simulink model "sampleModel1701"  (R2023a)
settings: Solver=VariableStepAuto  StartTime=0.0  StopTime=10.0  RelTol=1e-3
libraries: hdlsllib x3, simulink x1
settings Model: Creator=user1  LastModifiedBy=user1

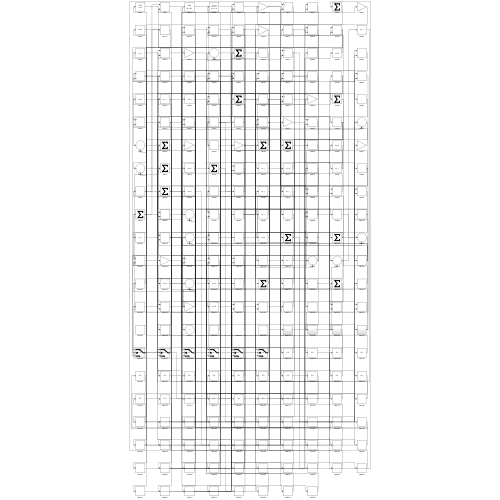
[thumbnail: Simulink's stored preview of the top-level diagram]
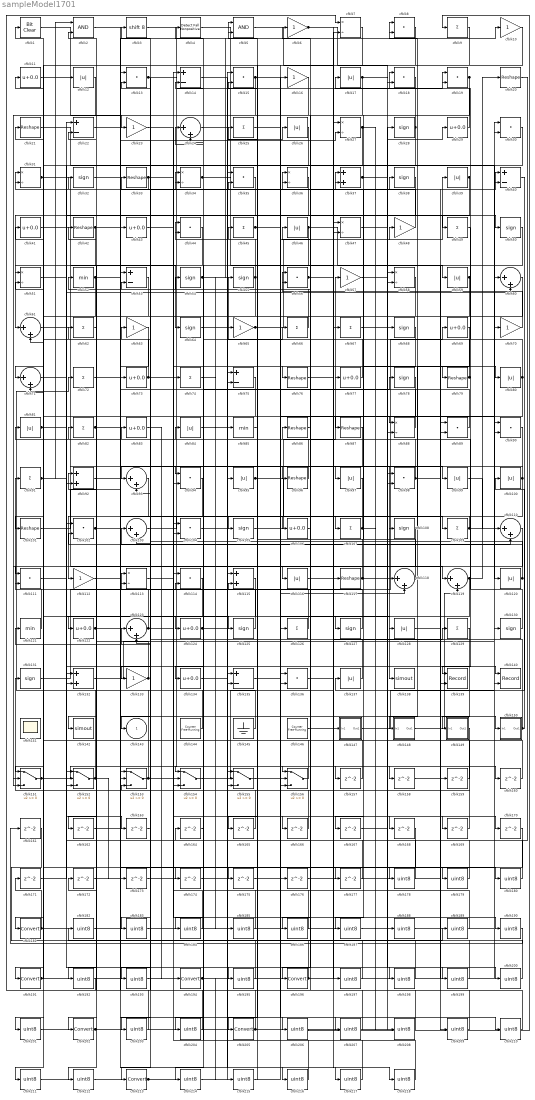
== system sampleModel1701 ==
  cfblk1 : simulink/Logic and Bit Operations/Bit Clear  iBit=0
      settings: LibrarySourceBlock=|
      | hdlsllib/Logic and Bit
      | Operations/Bit Clear
  cfblk{6,10,16,23,48,57,63,65,70,112,133} (11 alike) : Gain
  cfblk{12,17,26,39,46,59,80..81,84,95,97,99..100,116,120,128,137} (17 alike) : Abs  SaturateOnIntegerOverflow=off
  cfblk{20..21,33,42,76,79,86..87,96,101,117} (11 alike) : Reshape
  cfblk{8,13,15,18..19,30,35,44,56,89..90,94,98,102,104,111,114,136} (18 alike) : DotProduct  OutDataTypeStr=Inherit: Inherit via internal rule
  cfblk{24,60..61,71,93,103,110,118..119,123} (10 alike) : Sum  Inputs=|++
  cfblk{28,32,38,50,54..55,64,68,78,105,108,125,127,130..131} (15 alike) : Signum
  cfblk{11,29,41,43,69,73,77,83,106,122,124,134} (12 alike) : Bias  Bias=0.0  SaturateOnIntegerOverflow=off
  cfblk{9,25,45,49,62,66..67,72,74,82,91,107,109,126,129} (15 alike) : Sum  Inputs=+
  cfblk{7,27,31,34,36,47,51,58,88,113} (10 alike) : Product  Inputs=*/  RndMeth=Zero  SaturateOnIntegerOverflow=on
  cfblk{37,92,115,132} (4 alike) : Sum
  cfblk121 : MinMax
  cfblk{14,22,40,53,75,135} (6 alike) : Sum  Inputs=+-
  cfblk138 : ToWorkspace  VariableName=simout  SaveFormat=Timeseries  SampleTime=-1
  cfblk139 : Record  FileSettingsInternal="{\"entries\":[{\"content\":{\"excelSettings\":{\"content\":{},\"type\":\"Streamout.ExcelSettings\"}},\"type\":\"Streamout.FileSettingStorage\",\"uuid\":\"\"}],\"packageUris\":[\"http:\\/\\/schema.mathworks.com\\/mf0\\/streamout_blocks\\/R2020a\"],\"version\":\"1.0\"}"  Layout=[1 1]  SignalsInternal="{\"entries\":[{\"content\":{\"signals\":[{\"content\":{\"blockPath\":[],\"dimensions\":[1],\"domain\":\"\",\"lineColor\":\"#a2142f\",\"plots\":[1],\"port\":1,\"signalID\":3074,\"signalName\":\"XY Graph:1\"},\"type\":\"RecordBlkView.Signal\",\"uuid\":\"\"},{\"content\":{\"blockPath\":[],\"dimensions\":[1],\"domain\":\"\",\"lineColor\":\"#139fff\",\"plots\":[1],\"port\":2,\"signalID\":3077,\"signalName\":\"XY Graph:2\"},\"type\":\"RecordBlkView.Signal\",\"uuid\":\"\"}]},\"type\":\"RecordBlkView.InputSignals\",\"uuid\":\"\"}],\"packageUris\":[\"http:\\/\\/schema.mathworks.com\\/mf0\\/streamout_blocks\\/R2020a\"],\"version\":\"1.0\"}"  VisualizationBindings="{\"xyplotplugin\":{\"info\":[{\"series\":[{\"bindingParametersList\":[{\"parameter\":\"X-Axis\",\"signalID\":3074,\"signalName\":\"XY Graph:1\"},{\"parameter\":\"Y-Axis\",\"signalID\":3077,\"signalName\":\"XY Graph:2\"}],\"seriesID\":48839}],\"subplotID\":1}]}}"  CompatibilityTag=XY  st=-1
  cfblk140 : Record  FileSettingsInternal="{\"entries\":[{\"content\":{\"excelSettings\":{\"content\":{},\"type\":\"Streamout.ExcelSettings\"}},\"type\":\"Streamout.FileSettingStorage\",\"uuid\":\"\"}],\"packageUris\":[\"http:\\/\\/schema.mathworks.com\\/mf0\\/streamout_blocks\\/R2020a\"],\"version\":\"1.0\"}"  Layout=[1 1]  SignalsInternal="{\"entries\":[{\"content\":{\"signals\":[{\"content\":{\"blockPath\":[],\"dimensions\":[1],\"domain\":\"\",\"lineColor\":\"#a2142f\",\"plots\":[1],\"port\":1,\"signalID\":3082,\"signalName\":\"XY Graph:1\"},\"type\":\"RecordBlkView.Signal\",\"uuid\":\"\"},{\"content\":{\"blockPath\":[],\"dimensions\":[1],\"domain\":\"\",\"lineColor\":\"#139fff\",\"plots\":[1],\"port\":2,\"signalID\":3085,\"signalName\":\"XY Graph:2\"},\"type\":\"RecordBlkView.Signal\",\"uuid\":\"\"}]},\"type\":\"RecordBlkView.InputSignals\",\"uuid\":\"\"}],\"packageUris\":[\"http:\\/\\/schema.mathworks.com\\/mf0\\/streamout_blocks\\/R2020a\"],\"version\":\"1.0\"}"  VisualizationBindings="{\"xyplotplugin\":{\"info\":[{\"series\":[{\"bindingParametersList\":[{\"parameter\":\"X-Axis\",\"signalID\":3082,\"signalName\":\"XY Graph:1\"},{\"parameter\":\"Y-Axis\",\"signalID\":3085,\"signalName\":\"XY Graph:2\"}],\"seriesID\":35612}],\"subplotID\":1}]}}"  CompatibilityTag=XY  st=-1
  cfblk141 : Scope
      settings: Floating=on
  cfblk142 : ToWorkspace  VariableName=simout  SaveFormat=Timeseries  SampleTime=-1
  cfblk144 : hdlsllib/Sources/Counter Free-Running  NumBits=16  tsamp=-1
  cfblk145 : Ground
  cfblk146 : hdlsllib/Sources/Counter Free-Running  NumBits=16  tsamp=-1
  cfblk147 : Subsystem
      settings: LibrarySourceBlock=|
      | hdlsllib/Ports &
      | Subsystems/Subsystem
  cfblk148 : Subsystem
      settings: LibrarySourceBlock=|
      | hdlsllib/Ports &
      | Subsystems/Subsystem
  cfblk149 : Subsystem
      settings: LibrarySourceBlock=|
      | hdlsllib/Ports &
      | Subsystems/Subsystem
  cfblk150 : Subsystem
      settings: LibrarySourceBlock=|
      | hdlsllib/Ports &
      | Subsystems/Subsystem
  cfblk{151..156} (6 alike) : Switch  SaturateOnIntegerOverflow=off  InputSameDT=off
  cfblk{157..177} (21 alike) : Delay  SampleTime=1
  cfblk{178..180,182..190,192..193,195,197..201,203..204,206..212,214..218} (34 alike) : DataTypeConversion  OutDataTypeStr=uint8  SaturateOnIntegerOverflow=off  RndMeth=Floor
  cfblk{181,191,194,196,202,205,213} (7 alike) : DataTypeConversion  SaturateOnIntegerOverflow=off  RndMeth=Floor
  cfblk2 : Logic  AllPortsSameDT=off  OutDataTypeStr=boolean
  cfblk3 : ArithShift  BitShiftNumber=8
  cfblk4 : hdlsllib/Logic and Bit Operations/Detect Fall Nonpositive  vinit=0  OutDataTypeStr=boolean
  cfblk5 : Logic  AllPortsSameDT=off  OutDataTypeStr=boolean
  cfblk52 : MinMax
  cfblk85 : MinMax
  cfblk143 : Outport  VectorParamsAs1DForOutWhenUnconnected=off
  wires:
  cfblk79/1 -> cfblk55/1, cfblk8/1
  cfblk93/1 -> cfblk112/1
  cfblk74/1 -> cfblk85/1
  cfblk61/1 -> cfblk138/1
  cfblk99/1 -> cfblk110/1
  cfblk3/1 -> cfblk156/1
  cfblk80/1 -> cfblk17/1, cfblk94/1, cfblk212/1
  cfblk41/1 -> cfblk119/1
  cfblk130/1 -> cfblk84/1
  cfblk144/1 -> cfblk92/1
  cfblk54/1 -> cfblk10/1, cfblk76/1, cfblk185/1
  cfblk9/1 -> cfblk205/1
  cfblk40/1 -> cfblk137/1
  cfblk131/1 -> cfblk69/1
  cfblk36/1 -> cfblk61/1
  cfblk137/1 -> cfblk34/1
  cfblk85/1 -> cfblk5/1
  cfblk105/1 -> cfblk57/1
  cfblk152/1 -> cfblk72/1, cfblk173/1
  cfblk5/1 -> cfblk117/1
  cfblk88/1 -> cfblk77/1
  cfblk100/1 -> cfblk93/1, cfblk175/1
  cfblk133/1 -> cfblk62/1, cfblk121/1
  cfblk28/1 -> cfblk23/1, cfblk111/1
  cfblk149/1(Out1) -> cfblk131/1
  cfblk76/1 -> cfblk38/1
  cfblk50/1 -> cfblk134/1
  cfblk56/1 -> cfblk116/1, cfblk88/2
  cfblk145/1 -> cfblk21/1
  cfblk150/1(Out1) -> cfblk33/1, cfblk100/1
  cfblk146/1 -> cfblk147/1(In1)
  cfblk124/1 -> cfblk44/1, cfblk166/1
  cfblk33/1 -> cfblk31/2, cfblk35/2, cfblk203/1
  cfblk108/1 -> cfblk18/1, cfblk151/3
  cfblk101/1 -> cfblk36/1
  cfblk87/1 -> cfblk143/1
  cfblk147/1(Out1) -> cfblk119/2
  cfblk59/1 -> cfblk98/2, cfblk167/1, cfblk184/1
  cfblk91/1 -> cfblk41/1, cfblk12/1, cfblk60/2
  cfblk107/1 -> cfblk106/1, cfblk188/1
  cfblk92/1 -> cfblk78/1
  cfblk6/1 -> cfblk58/1, cfblk218/1
  cfblk153/1 -> cfblk52/1, cfblk177/1
  cfblk151/1 -> cfblk154/1, cfblk163/1
  cfblk103/1 -> cfblk108/1
  cfblk117/1 -> cfblk28/1, cfblk45/1
  cfblk125/1 -> cfblk113/1
  cfblk119/1 -> cfblk151/1, cfblk20/1
  cfblk35/1 -> cfblk75/2
  cfblk94/1 -> cfblk122/1
  cfblk31/1 -> cfblk64/1, cfblk49/1
  cfblk1/1 -> cfblk73/1
  cfblk111/1 -> cfblk140/1
  cfblk126/1 -> cfblk32/1
  cfblk98/1 -> cfblk11/1, cfblk170/1
  cfblk10/1 -> cfblk156/2
  cfblk48/1 -> cfblk3/1
  cfblk21/1 -> cfblk120/1
  cfblk49/1 -> cfblk139/1
  cfblk136/1 -> cfblk129/1
  cfblk4/1 -> cfblk67/1
  cfblk132/1 -> cfblk70/1
  cfblk123/1 -> cfblk81/1, cfblk190/1
  cfblk32/1 -> cfblk105/1
  cfblk122/1 -> cfblk5/2, cfblk8/2
  cfblk26/1 -> cfblk93/2
  cfblk16/1 -> cfblk181/1
  cfblk148/1(Out1) -> cfblk130/1
  cfblk156/1 -> cfblk113/2
  cfblk38/1 -> cfblk92/2
  cfblk7/1 -> cfblk191/1
  cfblk115/1 -> cfblk213/1
  cfblk65/1 -> cfblk39/1, cfblk88/1
  cfblk77/1 -> cfblk34/2
  cfblk52/1 -> cfblk27/2, cfblk61/2
  cfblk29/1 -> cfblk19/1
  cfblk43/1 -> cfblk74/1
  cfblk47/1 -> cfblk68/1
  cfblk83/1 -> cfblk194/1
  cfblk73/1 -> cfblk79/1, cfblk51/2
  cfblk34/1 -> cfblk50/1, cfblk126/1
  cfblk128/1 -> cfblk40/1
  cfblk129/1 -> cfblk149/1(In1)
  cfblk42/1 -> cfblk71/1, cfblk199/1
  cfblk12/1 -> cfblk71/2
  cfblk58/1 -> cfblk97/1
  cfblk55/1 -> cfblk132/2, cfblk44/2
  cfblk46/1 -> cfblk139/2, cfblk152/3, cfblk90/2, cfblk154/3
  cfblk39/1 -> cfblk103/2, cfblk51/1
  cfblk112/1 -> cfblk136/2
  cfblk51/1 -> cfblk102/1
  cfblk69/1 -> cfblk148/1(In1)
  cfblk109/1 -> cfblk60/1, cfblk107/1
  cfblk45/1 -> cfblk128/1, cfblk40/2
  cfblk13/1 -> cfblk19/2, cfblk123/2
  cfblk11/1 -> cfblk43/1
  cfblk81/1 -> cfblk2/1, cfblk195/1
  cfblk71/1 -> cfblk125/1
  cfblk64/1 -> cfblk99/1
  cfblk37/1 -> cfblk29/1, cfblk59/1
  cfblk154/1 -> cfblk47/2
  cfblk78/1 -> cfblk127/1
  cfblk70/1 -> cfblk56/1
  cfblk66/1 -> cfblk42/1
  cfblk27/1 -> cfblk152/2, cfblk208/1
  cfblk104/1 -> cfblk66/1
  cfblk120/1 -> cfblk31/1, cfblk82/1, cfblk102/2
  cfblk110/1 -> cfblk142/1
  cfblk18/1 -> cfblk133/1
  cfblk82/1 -> cfblk153/1, cfblk217/1
  cfblk95/1 -> cfblk109/1, cfblk37/1, cfblk48/1
  cfblk53/1 -> cfblk202/1
  cfblk19/1 -> cfblk96/1, cfblk87/1
  cfblk134/1 -> cfblk26/1
  cfblk127/1 -> cfblk25/1
  cfblk121/1 -> cfblk91/1
  cfblk106/1 -> cfblk36/2
  cfblk63/1 -> cfblk153/2
  cfblk118/1 -> cfblk6/1, cfblk37/2
  cfblk15/1 -> cfblk101/1, cfblk118/2
  cfblk2/1 -> cfblk156/3
  cfblk102/1 -> cfblk124/1, cfblk150/1(In1), cfblk110/2
  cfblk17/1 -> cfblk151/2, cfblk180/1
  cfblk96/1 -> cfblk54/1
  cfblk8/1 -> cfblk18/2
  cfblk86/1 -> cfblk196/1
  cfblk67/1 -> cfblk80/1
  cfblk89/1 -> cfblk4/1
  cfblk84/1 -> cfblk157/1
  cfblk157/1 -> cfblk1/1
  cfblk113/1 -> cfblk158/1
  cfblk159/1 -> cfblk27/1
  cfblk25/1 -> cfblk160/1
  cfblk160/1 -> cfblk132/1
  cfblk62/1 -> cfblk162/1
  cfblk163/1 -> cfblk123/1
  cfblk20/1 -> cfblk164/1
  cfblk60/1 -> cfblk165/1
  cfblk165/1 -> cfblk103/1
  cfblk166/1 -> cfblk153/3
  cfblk23/1 -> cfblk168/1
  cfblk57/1 -> cfblk169/1
  cfblk169/1 -> cfblk13/1
  cfblk171/1 -> cfblk152/1
  cfblk172/1 -> cfblk35/1
  cfblk173/1 -> cfblk104/2
  cfblk90/1 -> cfblk174/1
  cfblk174/1 -> cfblk75/1
  cfblk175/1 -> cfblk118/1
  cfblk176/1 -> cfblk89/2
  cfblk177/1 -> cfblk56/2
  cfblk22/1 -> cfblk178/1
  cfblk178/1 -> cfblk63/1
  cfblk162/1 -> cfblk179/1
  cfblk179/1 -> cfblk22/1
  cfblk180/1 -> cfblk22/2
  cfblk181/1 -> cfblk171/1, cfblk94/2, cfblk140/2
  cfblk182/1 -> cfblk16/1
  cfblk114/1 -> cfblk183/1
  cfblk183/1 -> cfblk159/1
  cfblk184/1 -> cfblk114/1
  cfblk185/1 -> cfblk114/2
  cfblk30/1 -> cfblk186/1
  cfblk186/1 -> cfblk136/1
  cfblk68/1 -> cfblk187/1
  cfblk187/1 -> cfblk30/1
  cfblk188/1 -> cfblk30/2
  cfblk161/1 -> cfblk189/1
  cfblk189/1 -> cfblk15/1
  cfblk190/1 -> cfblk161/1
  cfblk191/1 -> cfblk111/2, cfblk154/2, cfblk47/1
  cfblk44/1 -> cfblk192/1
  cfblk192/1 -> cfblk7/1
  cfblk97/1 -> cfblk193/1
  cfblk193/1 -> cfblk7/2
  cfblk194/1 -> cfblk90/1, cfblk215/1
  cfblk195/1 -> cfblk83/1
  cfblk196/1 -> cfblk2/2, cfblk89/1
  cfblk116/1 -> cfblk197/1
  cfblk197/1 -> cfblk86/1
  cfblk155/1 -> cfblk198/1
  cfblk198/1 -> cfblk13/2
  cfblk199/1 -> cfblk155/1
  cfblk167/1 -> cfblk200/1
  cfblk200/1 -> cfblk155/2
  cfblk170/1 -> cfblk201/1
  cfblk201/1 -> cfblk155/3
  cfblk202/1 -> cfblk58/2, cfblk98/1, cfblk95/1
  cfblk203/1 -> cfblk53/1
  cfblk168/1 -> cfblk204/1
  cfblk204/1 -> cfblk53/2
  cfblk205/1 -> cfblk182/1, cfblk172/1
  cfblk72/1 -> cfblk206/1
  cfblk206/1 -> cfblk9/1
  cfblk24/1 -> cfblk207/1
  cfblk207/1 -> cfblk15/2
  cfblk208/1 -> cfblk24/1
  cfblk158/1 -> cfblk209/1
  cfblk209/1 -> cfblk24/2
  cfblk135/1 -> cfblk210/1
  cfblk210/1 -> cfblk46/1
  cfblk75/1 -> cfblk211/1
  cfblk211/1 -> cfblk135/1
  cfblk212/1 -> cfblk135/2
  cfblk213/1 -> cfblk176/1, cfblk65/1
  cfblk164/1 -> cfblk214/1
  cfblk214/1 -> cfblk115/1
  cfblk215/1 -> cfblk115/2
  cfblk14/1 -> cfblk216/1
  cfblk216/1 -> cfblk104/1
  cfblk217/1 -> cfblk14/1
  cfblk218/1 -> cfblk14/2

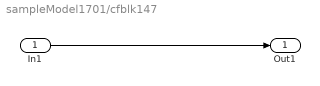
== system sampleModel1701/cfblk147 ==
  In1 : Inport
  Out1 : Outport
  wires:
  In1/1 -> Out1/1

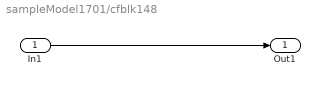
== system sampleModel1701/cfblk148 ==
  In1 : Inport
  Out1 : Outport
  wires:
  In1/1 -> Out1/1

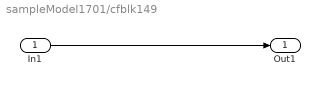
== system sampleModel1701/cfblk149 ==
  In1 : Inport
  Out1 : Outport
  wires:
  In1/1 -> Out1/1

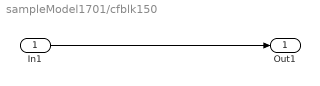
== system sampleModel1701/cfblk150 ==
  In1 : Inport
  Out1 : Outport
  wires:
  In1/1 -> Out1/1
